simulink model "car_model"  (R2024b)
settings: Solver=VariableStepAuto  StartTime=0.0  StopTime=10  RelTol=1e-3
values from neighbouring files (symbols this model uses):
  B = 10    [new-sim-workspace.mat]    (also in workspace-var-complete-jan.mat; workspace-vars.mat; workspace_var_dec_2024.mat; workspace_var_jan_2024.mat)
  C = 1.9    [new-sim-workspace.mat]    (also in workspace-var-complete-jan.mat; workspace-vars.mat; workspace_var_dec_2024.mat; workspace_var_jan_2024.mat)
  D = 1    [new-sim-workspace.mat]    (also in workspace-var-complete-jan.mat; workspace-vars.mat; workspace_var_dec_2024.mat; workspace_var_jan_2024.mat)
  g = 9.81    [new-sim-workspace.mat]    (also in workspace-var-complete-jan.mat; workspace-vars.mat; workspace_var_dec_2024.mat; workspace_var_jan_2024.mat)
  J_w = 0.5    [new-sim-workspace.mat]    (also in workspace-var-complete-jan.mat; workspace-vars.mat; workspace_var_dec_2024.mat; workspace_var_jan_2024.mat)
  M = 100    [new-sim-workspace.mat]    (also in workspace-var-complete-jan.mat; workspace-vars.mat; workspace_var_dec_2024.mat; workspace_var_jan_2024.mat)
  R = 0.5    [new-sim-workspace.mat]    (also in workspace-var-complete-jan.mat; workspace-vars.mat; workspace_var_dec_2024.mat; workspace_var_jan_2024.mat)
libraries: simulink x1, slpidlib x1
settings Model: Creator=kyle  LastModifiedBy=shykizzy

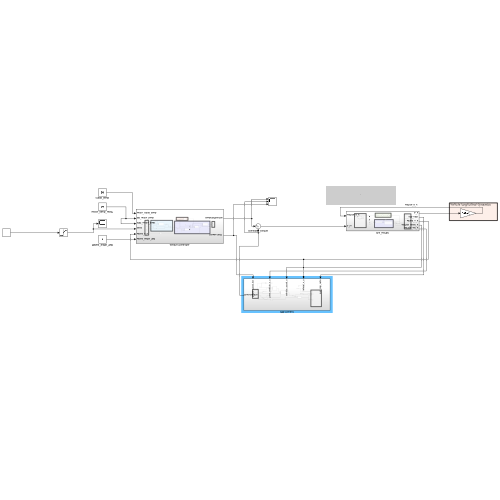
[thumbnail: Simulink's stored preview of the top-level diagram]
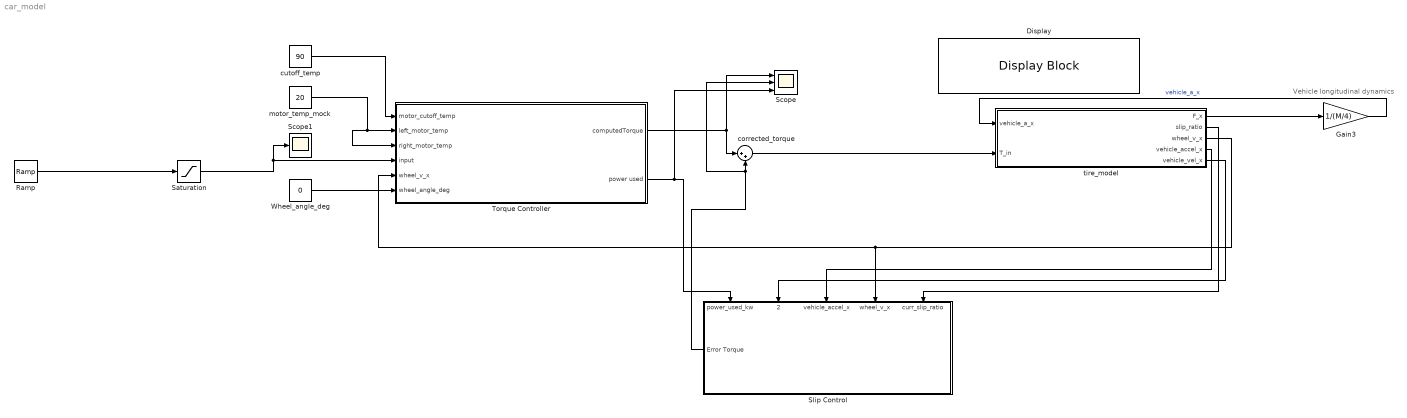
== system car_model ==
  note: Vehicle longitudinal dynamics
  Display : DisplayBlock  LabelPosition=Hide  Transparency=1
  Gain3 : Gain  Gain=1/(M/4)
  Ramp : simulink/Sources/Ramp  slope=1/2  start=1  InitialOutput=0
  Saturation : Saturate  UpperLimit=1  LowerLimit=0
  Scope : Scope  NumInputPorts=3
  Scope1 : Scope
  Slip Control : Subsystem
      settings: PortSchema="{\"entries\":[{\"content\":{\"sides\":[{\"content\":{\"connectorIds\":[\"Out1\"]},\"type\":\"ConnectorPlacement.EquallySpacedRectSide\",\"uuid\":\"3d629ccf-3120-465c-b95a-c1e856ea96ae\"},{\"content\":{\"side\":\"RIGHT\"},\"type\":\"ConnectorPlacement.EquallySpacedRectSide\",\"uuid\":\"39ac0bf8-cdbe-4e91-b33c-4b222cbdbfda\"},{\"content\":{\"connectorIds\":[\"In1\",\"In2\",\"In3\",\"In4\",\"In5\"],\"side\":\"TOP\"},\"type\":\"ConnectorPlacement.EquallySpacedRectSide\",\"uuid\":\"ede1119f-e1cb-4252-8f91-b266c29b68a7\"},{\"content\":{\"side\":\"BOTTOM\"},\"type\":\"ConnectorPlacement.EquallySpacedRectSide\",\"uuid\":\"e180508b-d381-4640-8659-6bcd533e6f5c\"}]},\"type\":\"ConnectorPlacement.EquallySpacedConnector\",\"uuid\":\"fb19f25d-abf5-424b-aa1b-adc6ce04aee5\"}],\"packageUris\":[\"http://schema.mathworks.com/mf0/Connector/R2020b\"],\"version\":\"1.0\"}"
  Torque Controller : Subsystem
  Wheel_angle_deg : Constant  Value=0
  corrected_torque : Sum  Inputs=|++
  cutoff_temp : Constant  Value=90
  motor_temp_mock : Constant  Value=20
  tire_model : Subsystem
  wires:
  tire_model/1(F_x) -> Gain3/1
  Gain3/1 -> tire_model/1(vehicle_a_x)  "vehicle_a_x"
  tire_model/2(slip_ratio) -> Slip Control/5(curr_slip_ratio)
  tire_model/3(wheel_v_x) -> Torque Controller/5(wheel_v_x), Slip Control/4(wheel_v_x)
  Ramp/1 -> Saturation/1
  Saturation/1 -> Scope1/1, Torque Controller/4(input)
  cutoff_temp/1 -> Torque Controller/1(motor_cutoff_temp)
  Wheel_angle_deg/1 -> Torque Controller/6(wheel_angle_deg)
  Torque Controller/1(computedTorque) -> corrected_torque/1, Scope/1
  corrected_torque/1 -> tire_model/2(T_in)
  motor_temp_mock/1 -> Torque Controller/2(left_motor_temp), Torque Controller/3(right_motor_temp)
  tire_model/4(vehicle_accel_x) -> Slip Control/3(vehicle_accel_x)
  tire_model/5(vehicle_vel_x) -> Slip Control/2(prev_vehicle_v_x)
  Torque Controller/2("power used ") -> Slip Control/1("power_used_kw "), Scope/3
  Slip Control/1(Error Torque) -> Scope/2, corrected_torque/2

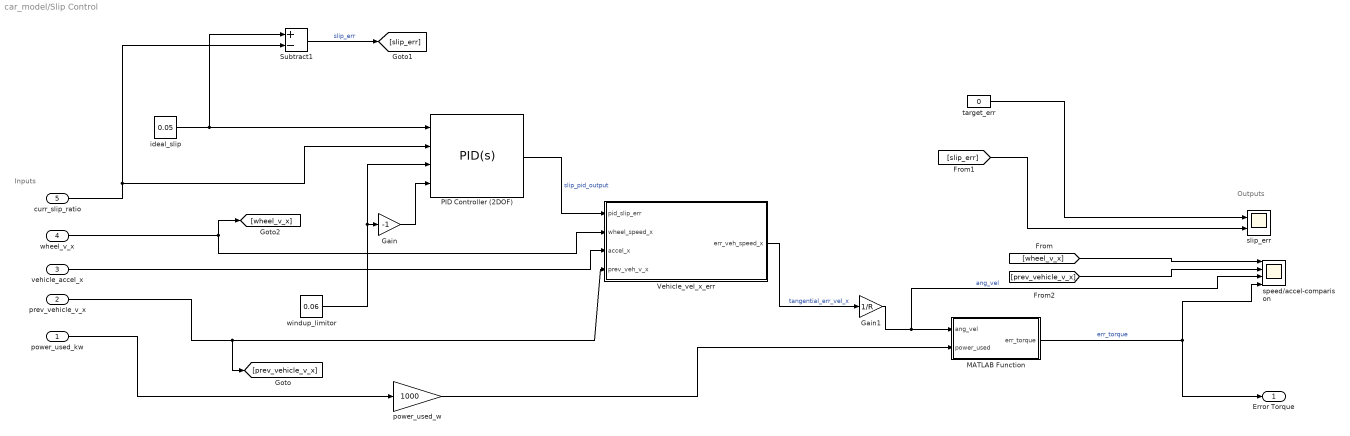
== system car_model/Slip Control ==
  note: Inputs
  note: Outputs
  "power_used_kw " : Inport
  prev_vehicle_v_x : Inport  Port=2
  vehicle_accel_x : Inport  Port=3
  wheel_v_x : Inport  Port=4
  curr_slip_ratio : Inport  Port=5
  Gain : Gain  Gain=-1
  Gain1 : Gain  Gain=1/R
  MATLAB Function : MATLAB Function  TreatAsAtomicUnit=on
  PID Controller (2DOF) : slpidlib/PID Controller (2DOF)  Controller=PID  Form=Parallel  TimeDomain=Continuous-time  UseExternalTs=off  SampleTime=-1  IntegratorMethod=Forward Euler  FilterMethod=Forward Euler  ControllerParametersSource=internal  P=1  I=0  UseKiTs=on  D=0  UseExternalDerivativeSource=off  N=10  UseFilter=on  b=1  c=1  TunerSelectOption=Transfer Function Based (PID Tuner App)  InitialConditionSource=internal  InitialConditionForIntegrator=0  InitialConditionForFilter=0  DifferentiatorICPrevScaledInput=0  ExternalReset=none  TrackingMode=off  Kt=1  LimitOutput=on  SatLimitsSource=external  UpperSaturationLimit=inf  LowerSaturationLimit=-inf  LinearizeAsGain=on  AntiWindupMode=clamping  Kb=1  LimitIntegrator=off  UpperIntegratorSaturationLimit=inf  LowerIntegratorSaturationLimit=-inf  POutMin=[]  POutMax=[]  IOutMin=[]  IOutMax=[]  DOutMin=[]  DOutMax=[]  NOutMin=[]  NOutMax=[]  bOutMin=[]  bOutMax=[]  cOutMin=[]  cOutMax=[]  SumOutMin=[]  SumOutMax=[]  SaturationOutMin=[]  SaturationOutMax=[]  PParamMin=[]  PParamMax=[]  IParamMin=[]  IParamMax=[]  DParamMin=[]  DParamMax=[]  NParamMin=[]  NParamMax=[]  bParamMin=[]  bParamMax=[]  cParamMin=[]  cParamMax=[]  KbParamMin=[]  KbParamMax=[]  KtParamMin=[]  KtParamMax=[]  KbOutMin=[]  KbOutMax=[]  KtOutMin=[]  KtOutMax=[]  IntegratorOutMin=[]  IntegratorOutMax=[]  FilterOutMin=[]  FilterOutMax=[]  SumI1OutMin=[]  SumI1OutMax=[]  SumI2OutMin=[]  SumI2OutMax=[]  SumI3OutMin=[]  SumI3OutMax=[]  SumI4OutMin=[]  SumI4OutMax=[]  SumDOutMin=[]  SumDOutMax=[]  Sum1OutMin=[]  Sum1OutMax=[]  Sum2OutMin=[]  Sum2OutMax=[]  Sum3OutMin=[]  Sum3OutMax=[]  DifferentiatorOutMin=[]  DifferentiatorOutMax=[]  FilterDiffOutCoefMin=[]  FilterDiffOutCoefMax=[]  ReciprocalOutMin=[]  ReciprocalOutMax=[]  SumDenOutMin=[]  SumDenOutMax=[]  SumNumOutMin=[]  SumNumOutMax=[]  DivideOutMin=[]  DivideOutMax=[]  UdiffTsProdOutMin=[]  UdiffTsProdOutMax=[]  NTsProdOutMin=[]  NTsProdOutMax=[]  UintegralTsProdOutMin=[]  UintegralTsProdOutMax=[]  UngainTsProdOutMin=[]  UngainTsProdOutMax=[]  ClampingZeroOutDataTypeStr=Inherit: Inherit via back propagation  ClampingZeroOutMin=[]  ClampingZeroOutMax=[]  FilterDenConstantOutDataTypeStr=Inherit: Inherit via back propagation  FilterDenConstantOutMin=[]  FilterDenConstantOutMax=[]  PCopyOutDataTypeStr=Inherit: Inherit via back propagation  PCopyOutMin=[]  PCopyOutMax=[]  NCopyOutDataTypeStr=Inherit: Inherit via back propagation  NCopyOutMin=[]  NCopyOutMax=[]  IntegratorContinuousStateAttributes=''  IntegratorStateMustResolveToSignalObject=off  IntegratorRTWStateStorageClass=Auto  FilterContinuousStateAttributes=''  FilterStateMustResolveToSignalObject=off  FilterRTWStateStorageClass=Auto  ParallelPVariant=InternalParameters  IdealPVariant=Disabled  IVariant=InternalParameters  DVariant=InternalParameters  bVariant=InternalParameters  cVariant=InternalParameters  IntegratorVariant=Continuous  SatVariant=External  AWVariant=ContClampingParallel  PCopyVariant=Disabled  TRVariant=Disabled  FdbkBlocksVariant=Forward  IdealPFdbkVariant=Disabled  SatFdbkVariant=Disabled  DerivativeFilterVariant=ContFilter  NVariant=InternalParameters  NCopyVariant=Disabled  FilterICVariant=InternalICsFilter  IntegratorICVariant=InternalICs  ExternalResetVariant=Disabled  TRSumVariant=Passthrough  SumFdbkVariant=Disabled  SumVariant=Sum_PID  TsampFilterVariant=InternalTs  TsampNgainVariant=Passthrough  TsampIntegralVariant=Disabled_SignalSpec  ExternalSaturationOutDataTypeStr=Inherit: Same as second input  DerivativeSourceVariant=ErrorSignal  PreIntVariant=InternalPreInt
  Subtract1 : Sum  Inputs=+-
  Vehicle_vel_x_err : MATLAB Function  TreatAsAtomicUnit=on
  ideal_slip : Constant  Value=0.05
  power_used_w : Gain  Gain=1000
  slip_err : Scope  NumInputPorts=2
  speed/accel-comparison : Scope  NumInputPorts=4
  target_err : Constant  Value=0
  windup_limitor : Constant  Value=0.06
  Error Torque : Outport
  wires:
  curr_slip_ratio/1 -> Subtract1/2, PID Controller (2DOF)/2
  ideal_slip/1 -> Subtract1/1, PID Controller (2DOF)/1
  PID Controller (2DOF)/1 -> Vehicle_vel_x_err/1(pid_slip_err)  "slip_pid_output"
  wheel_v_x/1 -> [wheel_v_x], Vehicle_vel_x_err/2(wheel_speed_x)
  Subtract1/1 -> [slip_err]  "slip_err"
  [slip_err] -> slip_err/2
  target_err/1 -> slip_err/1
  windup_limitor/1 -> PID Controller (2DOF)/3, Gain/1
  Gain/1 -> PID Controller (2DOF)/4
  vehicle_accel_x/1 -> Vehicle_vel_x_err/3(accel_x)
  prev_vehicle_v_x/1 -> [prev_vehicle_v_x], Vehicle_vel_x_err/4(prev_veh_v_x)
  [wheel_v_x] -> speed/accel-comparison/1
  [prev_vehicle_v_x] -> speed/accel-comparison/2
  Vehicle_vel_x_err/1(err_veh_speed_x) -> Gain1/1  "tangential_err_vel_x"
  Gain1/1 -> speed/accel-comparison/3, MATLAB Function/1(ang_vel)  "ang_vel"
  MATLAB Function/1(err_torque) -> Error Torque/1, speed/accel-comparison/4  "err_torque"
  "power_used_kw "/1 -> power_used_w/1
  power_used_w/1 -> MATLAB Function/2(power_used)

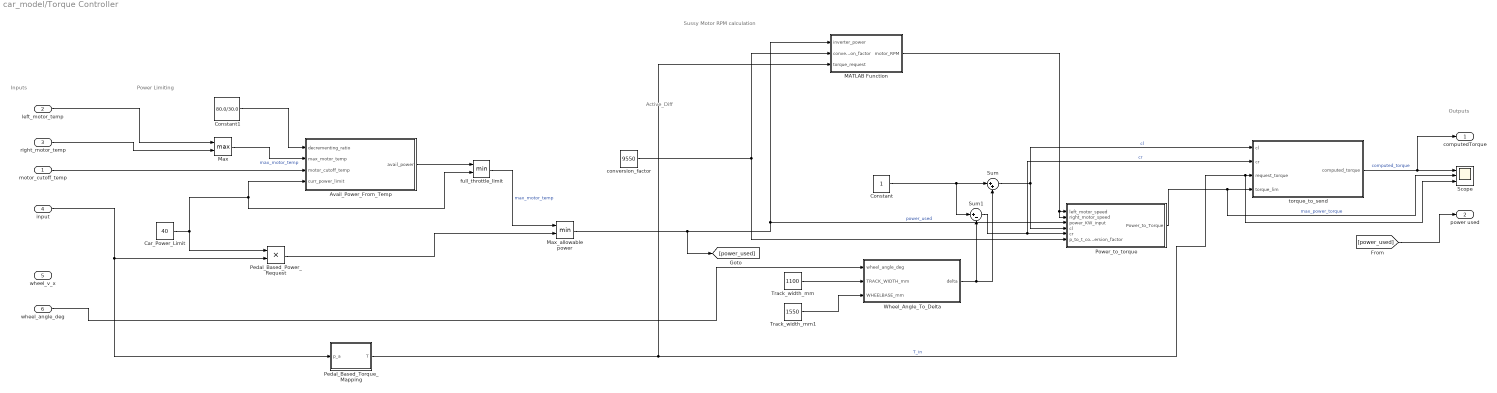
== system car_model/Torque Controller ==
  note: Active_Diff
  note: Inputs
  note: Outputs
  note: Power Limiting
  note: Sussy Motor RPM calculation
  motor_cutoff_temp : Inport
  left_motor_temp : Inport  Port=2
  right_motor_temp : Inport  Port=3
  input : Inport  Port=4
  wheel_v_x : Inport  Port=5
  wheel_angle_deg : Inport  Port=6
  Avail_Power_From_Temp : MATLAB Function  TreatAsAtomicUnit=on
  Car_Power_Limit : Constant  Value=40
  Constant : Constant
  Constant1 : Constant  Value=80.0/30.0
  MATLAB Function : MATLAB Function  TreatAsAtomicUnit=on
  Max : MinMax  Function=max  Inputs=2
  Max_allowable power : MinMax  Inputs=2
  Pedal_Based_Power_Request : Product
  Pedal_Based_Torque_Mapping : MATLAB Function  TreatAsAtomicUnit=on
  Power_to_torque : MATLAB Function  TreatAsAtomicUnit=on
  Scope : Scope  NumInputPorts=3
  Sum : Sum  Inputs=|++
  Sum1 : Sum  Inputs=|+-
  Track_width_mm : Constant  Value=1100
  Track_width_mm1 : Constant  Value=1550
  Wheel_Angle_To_Delta : MATLAB Function  TreatAsAtomicUnit=on
  conversion_factor : Constant  Value=9550
  full_throttle_limit : MinMax  Inputs=2
  torque_to_send : MATLAB Function  TreatAsAtomicUnit=on
  computedTorque : Outport
  "power used " : Outport  Port=2
  wires:
  input/1 -> Pedal_Based_Torque_Mapping/1(p_a), Pedal_Based_Power_Request/2
  left_motor_temp/1 -> Max/1
  right_motor_temp/1 -> Max/2
  motor_cutoff_temp/1 -> Avail_Power_From_Temp/3(motor_cutoff_temp)
  Car_Power_Limit/1 -> full_throttle_limit/2, Avail_Power_From_Temp/4(curr_power_limit), Pedal_Based_Power_Request/1
  Avail_Power_From_Temp/1(avail_power) -> full_throttle_limit/1
  full_throttle_limit/1 -> Max_allowable power/1  "max_motor_temp"
  Pedal_Based_Power_Request/1 -> Max_allowable power/2
  wheel_angle_deg/1 -> Wheel_Angle_To_Delta/1(wheel_angle_deg)
  Track_width_mm/1 -> Wheel_Angle_To_Delta/2(TRACK_WIDTH_mm)
  Track_width_mm1/1 -> Wheel_Angle_To_Delta/3(WHEELBASE_mm)
  Wheel_Angle_To_Delta/1(delta) -> Sum1/2, Sum/2
  Constant/1 -> Sum1/1, Sum/1
  Sum/1 -> Power_to_torque/4(cl), torque_to_send/1(cl)  "cl"
  Sum1/1 -> Power_to_torque/5(cr), torque_to_send/2(cr)  "cr"
  conversion_factor/1 -> Power_to_torque/6(p_to_t_conversion_factor), MATLAB Function/2(conversion_factor)
  Max_allowable power/1 -> [power_used], MATLAB Function/1(inverter_power), Power_to_torque/3(power_KW_input)  "power_used"
  Pedal_Based_Torque_Mapping/1(T) -> MATLAB Function/3(torque_request), Scope/3, torque_to_send/3(request_torque)  "T_in"
  MATLAB Function/1(motor_RPM) -> Power_to_torque/2(right_motor_speed), Power_to_torque/1(left_motor_speed)
  Power_to_torque/1(Power_to_Torque) -> Scope/2, torque_to_send/4(torque_lim)  "max_power_torque"
  torque_to_send/1(computed_torque) -> Scope/1, computedTorque/1  "computed_torque"
  Max/1 -> Avail_Power_From_Temp/2(max_motor_temp)  "max_motor_temp"
  Constant1/1 -> Avail_Power_From_Temp/1(decrementing_ratio)
  [power_used] -> "power used "/1

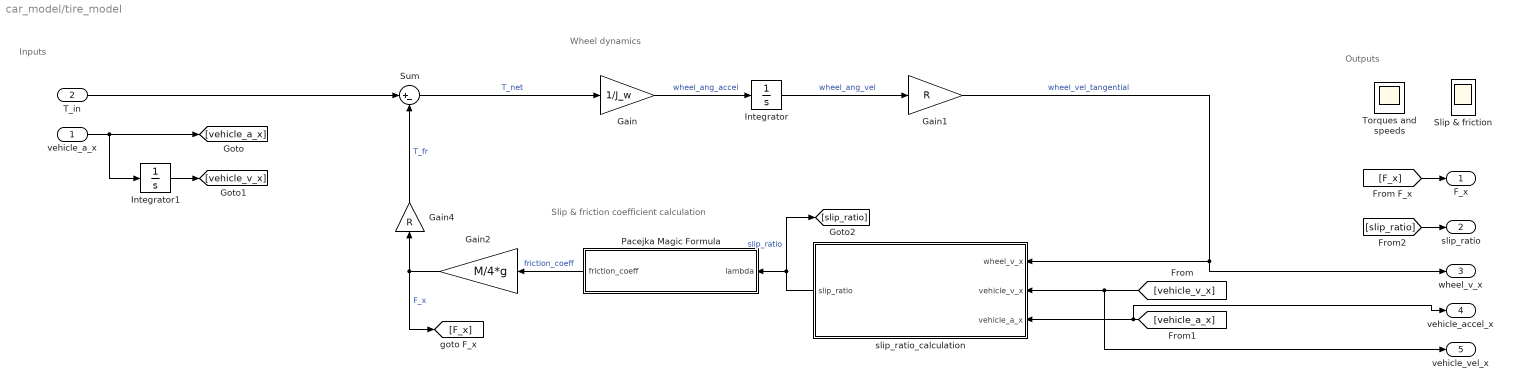
== system car_model/tire_model ==
  note: Inputs
  note: Slip & friction coefficient calculation
  note: Wheel dynamics
  note: Outputs
  vehicle_a_x : Inport
  T_in : Inport  Port=2
  Gain : Gain  Gain=1/J_w
  Gain1 : Gain  Gain=R
  Gain2 : Gain  Gain=M/4*g
  Gain4 : Gain  Gain=R
  Integrator : Integrator
  Integrator1 : Integrator
  Pacejka Magic Formula : MATLAB Function  TreatAsAtomicUnit=on
  Slip & friction : Scope
      settings: Floating=on
  Sum : Sum  Inputs=|+-
  Torques and speeds : Scope
      settings: Floating=on
  slip_ratio_calculation : MATLAB Function  TreatAsAtomicUnit=on
  F_x : Outport
  slip_ratio : Outport  Port=2
  wheel_v_x : Outport  Port=3
  vehicle_accel_x : Outport  Port=4
  vehicle_vel_x : Outport  Port=5
  wires:
  Sum/1 -> Gain/1  "T_net"
  Gain1/1 -> wheel_v_x/1, slip_ratio_calculation/1(wheel_v_x)  "wheel_vel_tangential"
  Integrator/1 -> Gain1/1  "wheel_ang_vel"
  Gain4/1 -> Sum/2  "T_fr"
  Gain/1 -> Integrator/1  "wheel_ang_accel"
  slip_ratio_calculation/1(slip_ratio) -> Pacejka Magic Formula/1(lambda), [slip_ratio]  "slip_ratio"
  T_in/1 -> Sum/1
  vehicle_a_x/1 -> Integrator1/1, [vehicle_a_x]
  Integrator1/1 -> [vehicle_v_x]
  [vehicle_v_x] -> vehicle_vel_x/1, slip_ratio_calculation/2(vehicle_v_x)
  [vehicle_a_x] -> vehicle_accel_x/1, slip_ratio_calculation/3(vehicle_a_x)
  [F_x] -> F_x/1
  [slip_ratio] -> slip_ratio/1
  Gain2/1 -> [F_x], Gain4/1  "F_x"
  Pacejka Magic Formula/1(friction_coeff) -> Gain2/1  "friction_coeff"

== matlab function car_model/Slip Control/MATLAB Function ==
  data: ang_vel input; power_used input; err_torque output
function err_torque = fcn(ang_vel, power_used)

% originally the plan to convert longitudinal vehicle speed to motor torque
% then differeniate to get angular acceleration then use t = m * a (the
% reason we dont multiple by R is because to go from longitudinal vel to
% ang vel we need to divide by R thus the simplified formula would just to
% be to cancel that with the multiplication with Radius to get torque
% however the the differentiation introduced alot of instability to the
% system which was becoming very difficult to stabilize through noise
% filtering and PID tuning 

% the plan here is to convert longitudinal velocity into angular velocity
% then use the formula T =  P / w to solve for torque  where P is the power
%  

small_epsilon = 0.1;
max_err_torque = 90; 


if(ang_vel <= 5)
    err_torque = 0;
else 
    err_torque = power_used / (ang_vel + small_epsilon) ;
end 

err_torque = max(min(err_torque, max_err_torque), -max_err_torque)

== matlab function car_model/tire_model/Pacejka Magic Formula ==
  data: lambda input double size=1; friction_coeff output double size=1; B parameter double size=1; C parameter double size=1; D parameter double size=1; E parameter double size=1
function friction_coeff = fcn(lambda, B, C, D, E)

friction_coeff = D*sin(C*atan(B*lambda -  E*(B*lambda - atan(B*lambda))));

== matlab function car_model/tire_model/slip_ratio_calculation ==
  data: wheel_v_x input; slip_ratio output; vehicle_v_x input; TOL parameter; vehicle_a_x input
function slip_ratio = fcn(wheel_v_x, vehicle_v_x, TOL, vehicle_a_x)
% This is derived from pg. 100 of Rajamani - Vehicle Dynamics and Control
% (2006)

if vehicle_a_x >= 0
    slip_ratio = (wheel_v_x- vehicle_v_x)/(wheel_v_x + TOL);
else
    slip_ratio = (wheel_v_x - vehicle_v_x)/(vehicle_v_x + TOL);
end

== matlab function car_model/Torque Controller/Avail_Power_From_Temp ==
  data: decrementing_ratio input; max_motor_temp input; avail_power output; motor_cutoff_temp input; curr_power_limit input
function avail_power = fcn( decrementing_ratio,max_motor_temp, ...
    motor_cutoff_temp, curr_power_limit)

avail_power = curr_power_limit;

if (max_motor_temp - motor_cutoff_temp) >= 30.0
    avail_power = 0.0;
elseif max_motor_temp > motor_cutoff_temp
    avail_power = curr_power_limit - ...
    (max_motor_temp - motor_cutoff_temp) * ...
    decrementing_ratio;
end

== matlab function car_model/Slip Control/Vehicle_vel_x_err ==
  data: pid_slip_err input; err_veh_speed_x output; wheel_speed_x input; accel_x input; prev_veh_v_x input
function err_veh_speed_x = fcn(pid_slip_err, wheel_speed_x, accel_x, ...
    prev_veh_v_x)
 

% formula used for calcualtion is slip = 
% (wheel_speed - vehicle_speed)/(vehicle or wheel speed depending on acel)
% we'll use the same calculation calulcation to calculate an error vehicle
% speed.. this will then need to be converted to an error torque

% when postively accelrating the tires tries spin faster than the car vel thus 
% we calculate slip with wheel speed as denom 
% if negatively accelerating the tire tries to spin slower than the vehicle
% thus vehicle velocity is used as denom  

small_epsilon = 0.1;

max_err= 100;

if(accel_x >= 0 )
    err_veh_speed_x = wheel_speed_x  - pid_slip_err * ...
    (wheel_speed_x + small_epsilon);
else
    err_veh_speed_x = wheel_speed_x - pid_slip_err * ...
    (prev_veh_v_x + small_epsilon);

    err_veh_speed_x = max(min(err_veh_speed_x, max_err), -max_err);

end

== matlab function car_model/Torque Controller/torque_to_send ==
  data: computed_torque output; cl input; cr input; request_torque input; torque_lim input
% this block should theoritically not do anything as of now because of the
% way motor speed was calculate (the output of maxPower_to_Torque is going
% to be requested torque as of now)

function computed_torque = fcn(cl, cr, request_torque, torque_lim)

% will be the same for now 
torque_left_nm = request_torque * cl; 
torque_right_nm = request_torque * cr; 
scale = 1.0; 

torque_req_max = max([torque_left_nm, torque_right_nm]);

if torque_req_max > torque_lim 
    scale = torque_lim / torque_req_max;
end 
computed_torque = torque_req_max * scale;

== matlab function car_model/Torque Controller/Wheel_Angle_To_Delta ==
  data: wheel_angle_deg input; TRACK_WIDTH_mm input; WHEELBASE_mm input; delta output
function delta = fcn(wheel_angle_deg, TRACK_WIDTH_mm, WHEELBASE_mm)

delta = TRACK_WIDTH_mm * tan(deg2rad(wheel_angle_deg)) / (2 * WHEELBASE_mm);

== matlab function car_model/Torque Controller/Power_to_torque ==
  data: left_motor_speed input; right_motor_speed input; power_KW_input input; cl input; Power_to_Torque output; cr input; p_to_t_conversion_factor input
function Power_to_Torque = fcn(left_motor_speed, right_motor_speed,power_KW_input, ...
    cl,cr, p_to_t_conversion_factor)

% taken directly from code .. standard motor torque charac eqn assumes
% torque is equally distributed between left and right wheel

% since our power limit torque is calcuated using requested torque if we
% use the name power to torque formula that we use in code we will always
% get half of the requested torque as the limit and there fore the output
% torque will be defaulted to the power limit... good thing is that this
% shows that the defaulting if power limit torque exceeded works bad thing
% is that we are straying away from our actual mathematical model...
% tentatively I have changed the calculation for power to torque from power
% limit to only account for 1 wheel as this is a one wheel model

Power_to_Torque = (p_to_t_conversion_factor * power_KW_input)/ ...
(left_motor_speed + 0.00001);

== matlab function car_model/Torque Controller/Pedal_Based_Torque_Mapping ==
  data: p_a input; T output
function T = fcn(p_a)

T = 90*p_a

== matlab function car_model/Torque Controller/MATLAB Function ==
  data: inverter_power input; conversion_factor input; torque_request input; motor_RPM output
function motor_RPM = fcn(inverter_power, conversion_factor, torque_request)

% kinda sus calculation but we need a way to calculate motor speed from
% torque... decided to use T = 9550 * P in KW / N in rpm 
% problem is the power_to_torque function just calculates using the same
% formula so essentially it will go back to the torque request 

motor_RPM = (inverter_power * conversion_factor) / (torque_request + 0.00001);
